simulink model "Simulation_CT"  (R2022a)
settings: Solver=VariableStepAuto  StartTime=0.0  StopTime=1  RelTol=1e-3
values from neighbouring files (symbols this model uses):
  K_d = 30 * diag([1 1 1 1 1 1])    [CT.m]
  K_p = 100 * diag([1 1 1 1 1 1])    [CT.m]
  max_tau = 100 * [1 1 1 1 1 1]    [CT.m]
undefined symbols (not defined in the file or in its folder): inertia, p560, q0, q_vel0
settings Model: Creator=Matteo Pettinari  LastModifiedBy=v
settings SolverCC: AlgebraicLoopSolver=TrustRegion
settings DebuggingCC: UnconnectedInputMsg=warning  UnconnectedOutputMsg=warning  UnconnectedLineMsg=warning  SFMachineParentedDataDiag=warning  ArithmeticOperatorsInVariantConditions=warning
settings SFSimCC: CustomCodeUndefinedFunction=UseInterfaceOnly

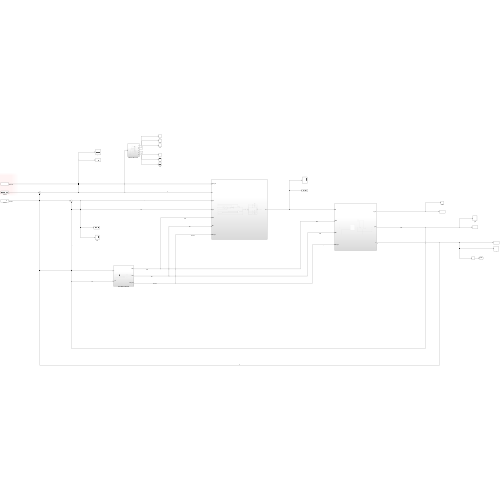
[thumbnail: Simulink's stored preview of the top-level diagram]
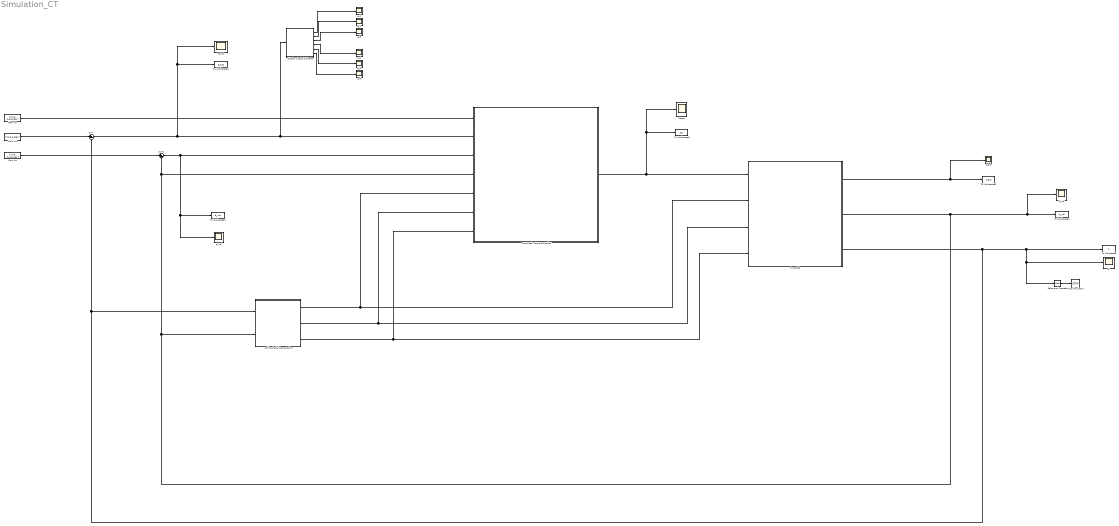
== system Simulation_CT ==
  "Computed Torque Controller " : Subsystem
  "Display single joint error " : Subsystem
  From ws : FromWorkspace  VariableName=[ time q_acc_des ]
  "From ws " : FromWorkspace  VariableName=[ time q_des ]
  "From ws " : FromWorkspace  VariableName=[ time q_vel_des ]
  Online Model Computation : Subsystem
  "Puma560 " : Subsystem
  Relational Operator : RelationalOperator  Operator=isNaN  OutDataTypeStr=boolean  InputSameDT=off
  Scope : Scope
  Stop Simulation : Stop
  Sum : Sum  Inputs=|+-
  Sum1 : Sum  Inputs=|+-
  To Workspace : ToWorkspace  VariableName=q  SaveFormat=Structure With Time  SampleTime=-1
  To Workspace1 : ToWorkspace  VariableName=q_vel  SaveFormat=Structure With Time  SampleTime=-1
  To Workspace2 : ToWorkspace  VariableName=q_acc  SaveFormat=Structure With Time  SampleTime=-1
  To Workspace3 : ToWorkspace  VariableName=e_pos  SaveFormat=Structure With Time  SampleTime=-1
  To Workspace4 : ToWorkspace  VariableName=e_vel  SaveFormat=Structure With Time  SampleTime=-1
  To Workspace6 : ToWorkspace  VariableName=tau  SaveFormat=Structure With Time  SampleTime=-1
  e_{1..6} (6 alike) : Scope
  "e_pos " : Scope
  e_vel : Scope
  q : Scope
  q_acc : Scope
  "q_vel " : Scope
  wires:
  "Puma560 "/3(q) -> Relational Operator/1, q/1, To Workspace/1, Sum/2, Online Model Computation/1(q)  "q"
  "Puma560 "/2(q_vel) -> Online Model Computation/2(q_vel), "Computed Torque Controller "/4(q_vel), Sum1/2, "q_vel "/1, To Workspace1/1  "q_vel"
  Online Model Computation/1(M(q)) -> "Computed Torque Controller "/5("M(q) "), "Puma560 "/2(M(q))  "M(q)"
  Online Model Computation/3(C(q,q_vel)) -> "Computed Torque Controller "/7(C(q,q_vel)), "Puma560 "/4(C(q,q_vel))  "C(q,q_vel)"
  Online Model Computation/2(G(q)) -> "Computed Torque Controller "/6("G(q) "), "Puma560 "/3(G(q))  "G(q)"
  Relational Operator/1 -> Stop Simulation/1
  Sum1/1 -> e_vel/1, To Workspace4/1, "Computed Torque Controller "/3(e_vel)  "e_vel"
  "Computed Torque Controller "/1(tau) -> To Workspace6/1, Scope/1, "Puma560 "/1(tau)
  From ws/1 -> "Computed Torque Controller "/1(q_acc_des)  "q_acc_des"
  "From ws "/1 -> Sum1/1  "q_vel_des"
  "From ws "/1 -> Sum/1  "q_des"
  "Puma560 "/1(q_acc) -> q_acc/1, To Workspace2/1
  "Display single joint error "/5(Out5) -> e_5/1
  "Display single joint error "/3(Out3) -> e_3/1
  Sum/1 -> "e_pos "/1, To Workspace3/1, "Display single joint error "/1(e), "Computed Torque Controller "/2(e)  "e"
  "Display single joint error "/6(Out6) -> e_6/1
  "Display single joint error "/4(Out4) -> e_4/1
  "Display single joint error "/1(Out1) -> e_1/1
  "Display single joint error "/2(Out2) -> e_2/1

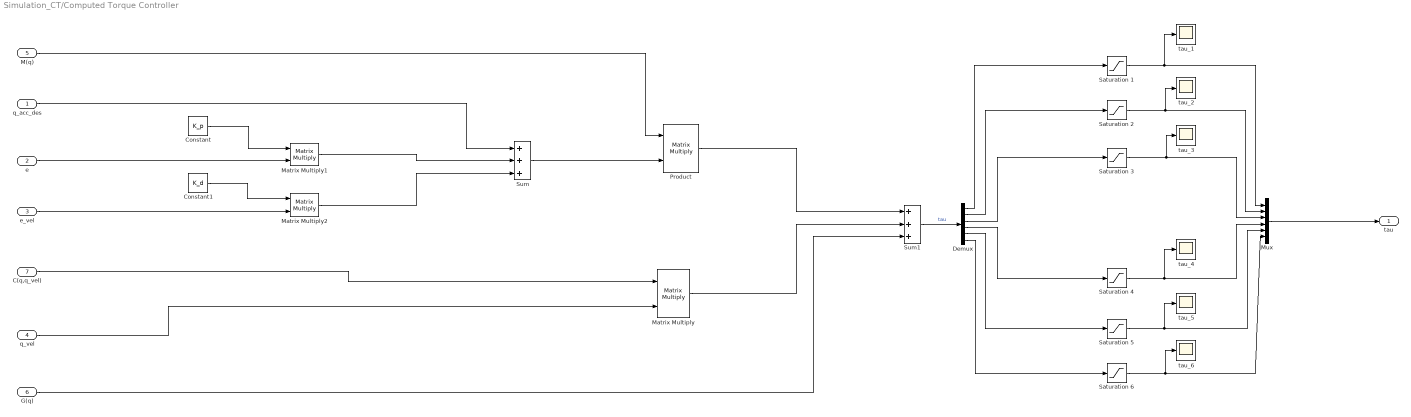
== system Simulation_CT/Computed Torque Controller  ==
  q_acc_des : Inport
  e : Inport  Port=2
  e_vel : Inport  Port=3
  q_vel : Inport  Port=4
  "M(q) " : Inport  Port=5
  "G(q) " : Inport  Port=6
  C(q,q_vel) : Inport  Port=7
  Constant : Constant  Value=K_p  VectorParams1D=off
  Constant1 : Constant  Value=K_d  VectorParams1D=off
  Demux : Demux  Outputs=6
  Matrix Multiply : Product  Multiplication=Matrix(*)
  Matrix Multiply1 : Product  Multiplication=Matrix(*)
  Matrix Multiply2 : Product  Multiplication=Matrix(*)
  Mux : Mux  Inputs=6
  Product : Product  Multiplication=Matrix(*)
  Saturation 1 : Saturate  UpperLimit=max_tau(1)  LowerLimit=-max_tau(1)
  Saturation 2 : Saturate  UpperLimit=max_tau(2)  LowerLimit=-max_tau(2)
  Saturation 3 : Saturate  UpperLimit=max_tau(3)  LowerLimit=-max_tau(3)
  Saturation 4 : Saturate  UpperLimit=max_tau(4)  LowerLimit=-max_tau(4)
  Saturation 5 : Saturate  UpperLimit=max_tau(5)  LowerLimit=-max_tau(5)
  Saturation 6 : Saturate  UpperLimit=max_tau(6)  LowerLimit=-max_tau(6)
  Sum : Sum  Inputs=+++
  Sum1 : Sum  Inputs=+++
  tau_1 : Scope
  "tau_2 " : Scope
  tau_3 : Scope
  "tau_4 " : Scope
  tau_5 : Scope
  "tau_6 " : Scope
  tau : Outport  VectorParamsAs1DForOutWhenUnconnected=off
  wires:
  q_acc_des/1 -> Sum/1
  Saturation 1/1 -> tau_1/1, Mux/1
  e_vel/1 -> Matrix Multiply2/2
  "G(q) "/1 -> Sum1/3
  Sum/1 -> Product/2
  "M(q) "/1 -> Product/1
  C(q,q_vel)/1 -> Matrix Multiply/1
  q_vel/1 -> Matrix Multiply/2
  Matrix Multiply/1 -> Sum1/2
  Product/1 -> Sum1/1
  Sum1/1 -> Demux/1  "tau"
  Demux/1 -> Saturation 1/1
  Mux/1 -> tau/1
  Saturation 2/1 -> "tau_2 "/1, Mux/2
  Demux/2 -> Saturation 2/1
  Demux/3 -> Saturation 3/1
  Saturation 3/1 -> tau_3/1, Mux/3
  Demux/4 -> Saturation 4/1
  Saturation 4/1 -> "tau_4 "/1, Mux/4
  Demux/5 -> Saturation 5/1
  Saturation 5/1 -> tau_5/1, Mux/5
  Demux/6 -> Saturation 6/1
  Saturation 6/1 -> Mux/6, "tau_6 "/1
  Constant/1 -> Matrix Multiply1/1
  e/1 -> Matrix Multiply1/2
  Matrix Multiply1/1 -> Sum/2
  Constant1/1 -> Matrix Multiply2/1
  Matrix Multiply2/1 -> Sum/3

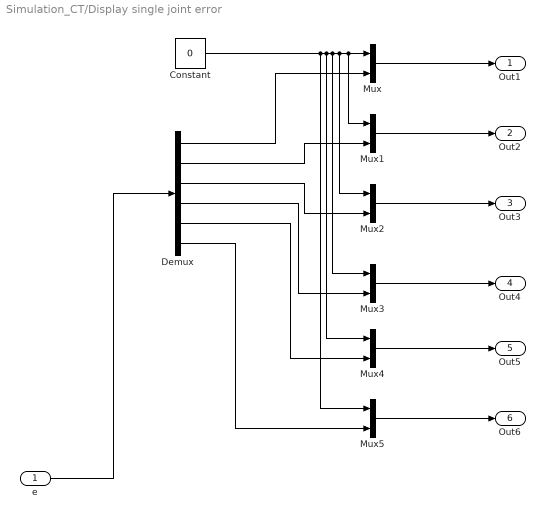
== system Simulation_CT/Display single joint error  ==
  e : Inport
  Constant : Constant  Value=0
  Demux : Demux  Outputs=6
  Mux{,1..5} (6 alike) : Mux  Inputs=2
  Out1 : Outport  VectorParamsAs1DForOutWhenUnconnected=off
  Out2 : Outport  Port=2  VectorParamsAs1DForOutWhenUnconnected=off
  Out3 : Outport  Port=3  VectorParamsAs1DForOutWhenUnconnected=off
  Out4 : Outport  Port=4  VectorParamsAs1DForOutWhenUnconnected=off
  Out5 : Outport  Port=5  VectorParamsAs1DForOutWhenUnconnected=off
  Out6 : Outport  Port=6  VectorParamsAs1DForOutWhenUnconnected=off
  wires:
  Mux3/1 -> Out4/1
  Constant/1 -> Mux5/1, Mux4/1, Mux3/1, Mux2/1, Mux1/1, Mux/1
  Demux/5 -> Mux4/2
  Demux/4 -> Mux3/2
  Mux2/1 -> Out3/1
  Demux/1 -> Mux/2
  Demux/2 -> Mux1/2
  Mux4/1 -> Out5/1
  Demux/3 -> Mux2/2
  Demux/6 -> Mux5/2
  Mux5/1 -> Out6/1
  Mux1/1 -> Out2/1
  Mux/1 -> Out1/1
  e/1 -> Demux/1

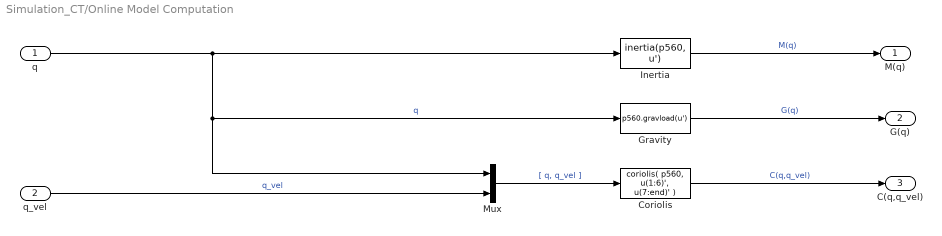
== system Simulation_CT/Online Model Computation ==
  q : Inport
  q_vel : Inport  Port=2
  Coriolis : MATLABFcn  MATLABFcn=coriolis( p560, u(1:6)', u(7:end)' )  Output1D=off
  Gravity : MATLABFcn  MATLABFcn=p560.gravload(u')  Output1D=off
  Inertia : MATLABFcn  MATLABFcn=inertia(p560, u')  Output1D=off
  Mux : Mux  Inputs=2
  M(q) : Outport  VectorParamsAs1DForOutWhenUnconnected=off
  G(q) : Outport  Port=2  VectorParamsAs1DForOutWhenUnconnected=off
  C(q,q_vel) : Outport  Port=3  VectorParamsAs1DForOutWhenUnconnected=off
  wires:
  Coriolis/1 -> C(q,q_vel)/1  "C(q,q_vel)"
  Mux/1 -> Coriolis/1  "[ q, q_vel ]"
  q_vel/1 -> Mux/2  "q_vel"
  q/1 -> Inertia/1, Mux/1, Gravity/1  "q"
  Inertia/1 -> M(q)/1  "M(q)"
  Gravity/1 -> G(q)/1  "G(q)"

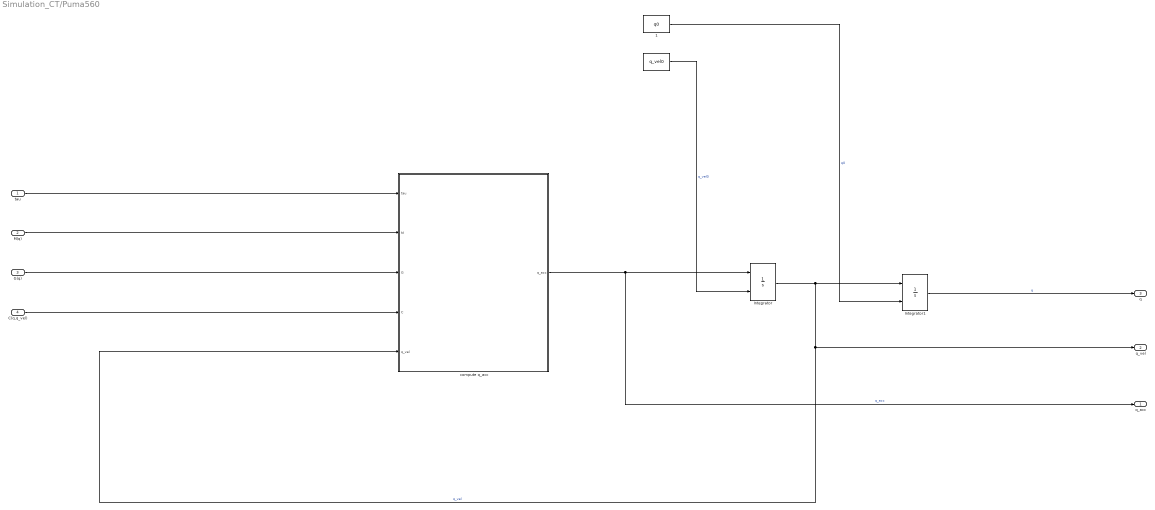
== system Simulation_CT/Puma560  ==
  tau : Inport
  M(q) : Inport  Port=2
  G(q) : Inport  Port=3
  C(q,q_vel) : Inport  Port=4
  " " : Constant  Value=q_vel0
  " 1" : Constant  Value=q0
  Integrator : Integrator  InitialConditionSource=external
  Integrator1 : Integrator  InitialConditionSource=external
  compute q_acc : MATLAB Function  TreatAsAtomicUnit=on
  q_acc : Outport  VectorParamsAs1DForOutWhenUnconnected=off
  q_vel : Outport  Port=2  VectorParamsAs1DForOutWhenUnconnected=off
  q : Outport  Port=3  VectorParamsAs1DForOutWhenUnconnected=off
  wires:
  " 1"/1 -> Integrator1/2  "q0"
  M(q)/1 -> compute q_acc/2(M)
  " "/1 -> Integrator/2  "q_vel0"
  compute q_acc/1(q_acc) -> q_acc/1, Integrator/1  "q_acc"
  Integrator/1 -> compute q_acc/5(q_vel), q_vel/1, Integrator1/1  "q_vel"
  G(q)/1 -> compute q_acc/3(G)
  tau/1 -> compute q_acc/1(tau)
  C(q,q_vel)/1 -> compute q_acc/4(C)
  Integrator1/1 -> q/1  "q"

== matlab function Simulation_CT/Puma560 /compute q_acc ==
  data: tau input; M input; G input; C input; q_vel input; q_acc output
%% *******************************************   compute_q_acc.m   *********************************************
% La funzione calcola l'accelerazione reale dei giunti dato in ingresso il modello del Puma560 e 
% l'ingresso da controllore tau.
%
% N.B.: Le forze di attrito F(q) son supposte nulle
%
%
% INPUT:
% - M(q)                                    : matrice del robot nella configurazione q(t)
% - C(q)                                    : matrice di Coriolis "
% - G(q)                                    : vettore gravità "
% - q_vel(t)                                : vel giunti vera ( moltiplica C(q,q_vel) )
% - tau                                     : computed torque da controllore
%
% OUTPUT:
% - q_acc(t)                                : accelerazione reale dei giunti



function q_acc = compute_q_acc( tau, M, G, C, q_vel)
    
    % Inversione della dinamica Lagrangiana Q = M(q)*q_acc + C(q,q_vel)*q_vel + G(q)
    q_acc = inv(M) * (tau - G' - C*q_vel );

end
